simulink model "Power_Systems_II_Simulation"  (R2022b)
settings: Solver=VariableStepAuto  StartTime=0.0  StopTime=4  RelTol=1e-3
libraries: spsGroundLib x5, spsVoltageMeasurementLib x3, spsThreePhaseFaultLib x1, spsCurrentMeasurementLib x1, spsDistributedParametersLineLib x1, spsThreePhaseSeriesRLCBranchLib x1, spsThreePhaseSourceLib x1, sps_lib x1
settings Model: Creator=USER  LastModifiedBy=USER

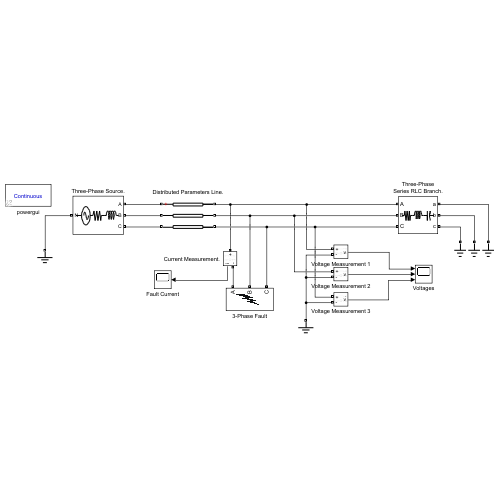
[thumbnail: Simulink's stored preview of the top-level diagram]
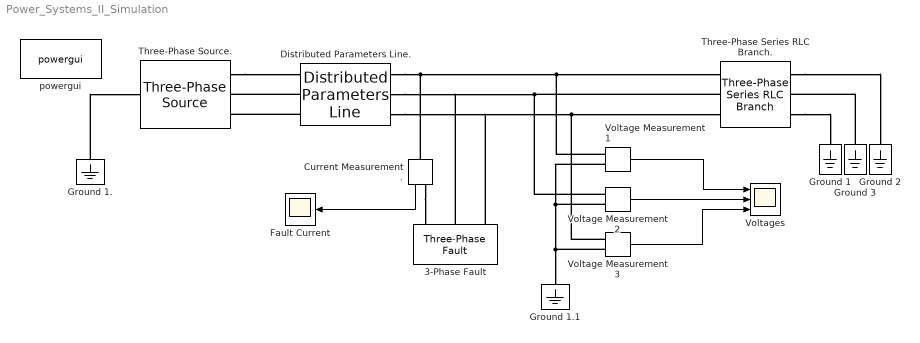
== system Power_Systems_II_Simulation ==
  3-Phase Fault : spsThreePhaseFaultLib/Three-Phase Fault  InitialStates=1  FaultA=on  FaultB=off  FaultC=off  GroundFault=on  SwitchTimes="[1  5]"  External=off  SwitchStatus=NaN  FaultResistance=0.01  GroundResistance=0.01  SnubberResistance=1e6  SnubberCapacitance=inf  Measurements=None
  Current Measurement. : spsCurrentMeasurementLib/Current Measurement  PhasorSimulation=off  OutputType=Complex  PSBequivalent=0
  Distributed Parameters Line. : spsDistributedParametersLineLib/Distributed Parameters Line  Phases=3  Length=10  Frequency=50  Resistance=[0.1 0.1]  Inductance=[0.3183 0.00095]  Capacitance=[0.00001 0.00001]  x1=[77.8287131632967 10973.8048950639 11040.6367185842;314.159265358979 314.159265358979 314.159265358979;-1.71456896003776 1.19594865444981 -0.369209675509595]  x2=[281.416313881128 4968.77740365391 8364.21694231392;314.159265358979 314.159265358979 314.159265358979;-0.928264752183291 2.28039663965508 -0.898944896122367]  x3=[78.9240246113386 59.1908510089468 99.800748397703;314.159265358979 314.159265358979 314.159265358979;-1.9368174494414 -0.00240562107416638 -0.495420267168485]  x4=[57.5363481374095 114.643353425724 27.3819360505492;314.159265358979 314.159265358979 314.159265358979;0.834085976351815 2.37283316623951 0.779404320473407]  x5=0.0178409640995099  V1=[77.83 1.097e+04 1.104e+04;314.2 314.2 314.2;-1.715 1.196 -0.3692]  V2=[281.4 4969 8364;314.2 314.2 314.2;-0.9283 2.28 -0.8989]  I1=[78.92 59.19 99.8;314.2 314.2 314.2;-1.937 -0.002406 -0.4954]  I2=[57.54 114.6 27.38;314.2 314.2 314.2;0.8341 2.373 0.7794]  nHarmo=1  Measurements=None  Decoupling=off  VsMag0=0  VrMag0=0  VsAngle0=0  VrAngle0=0  IsMag0=0  IrMag0=0  IsAngle0=0  IrAngle0=0
      settings: LibrarySourceBlock=sps_lib/Power Grid Elements/Distributed Parameters Line
  Fault Current : Scope
  Ground 1 : spsGroundLib/Ground  LConnTagsString=a
  Ground 1. : spsGroundLib/Ground  LConnTagsString=a
  Ground 1.1 : spsGroundLib/Ground  LConnTagsString=a
  Ground 2 : spsGroundLib/Ground  LConnTagsString=a
  Ground 3 : spsGroundLib/Ground  LConnTagsString=a
  Three-Phase Series RLC Branch. : spsThreePhaseSeriesRLCBranchLib/Three-Phase Series RLC Branch  LConnTagsString=A|B|C  RConnTagsString=A|B|C  BranchType=RLC  Resistance=3  Inductance=0.000795774  Capacitance=0.00001  Measurements=None
  Three-Phase Source. : spsThreePhaseSourceLib/Three-Phase Source  InternalConnection=Yn  VoltagePhases=off  Voltage=11000  PhaseAngle=0  Voltage_phases=[25e3 25e3 25e3]/sqrt(3)  PhaseAngles_phases=[0 -120 +120]  Frequency=50  NonIdealSource=on  SpecifyImpedance=off  Resistance=1  Inductance=0.000795774  ShortCircuitLevel=100e6  BaseVoltage=11000  XRratio=7  BusType=swing  Pref=10e3  Qref=0  Prefabc=[10e3, 10e3, 10e3]  Qrefabc=[0, 0, 0]  Qmin=-inf  Qmax=inf
  Voltage Measurement 1 : spsVoltageMeasurementLib/Voltage Measurement  PhasorSimulation=off  OutputType=Complex  PSBequivalent=0
  Voltage Measurement 2 : spsVoltageMeasurementLib/Voltage Measurement  PhasorSimulation=off  OutputType=Complex  PSBequivalent=0
  Voltage Measurement 3 : spsVoltageMeasurementLib/Voltage Measurement  PhasorSimulation=off  OutputType=Complex  PSBequivalent=0
  Voltages : Scope  NumInputPorts=3
  powergui : sps_lib/powergui  Priority=1  SimulationMode=Continuous  SampleTime=50e-6  frequency=60  Iterations=50  frequencyindice=50  Pbase=100e6  ErrMax=1e-4  UnitsV=kV  UnitsW=MW  buscounter=0  FunctionMessages=off  echomessages=off  EnableUseOfTLC=off  CurrentSourceSwitches=off  DisableSnubberDevices=off  DisableRonSwitches=off  DisableVfSwitches=off  DisplayEquations=off  AutomaticDiscreteSolvers=off  SolverType=Tustin/Backward Euler (TBE)  Interpol=off  ExternalGateDelay=off  methode=off  Ts=100  x0status=blocks  SPID=on  SwTol=0  HookPort=off  NonlinearTolerance=1e-4  nMaxIteration=100  ContinueOnMaxIteration=off  RestoreLinks=warning  ResistiveCurrentMeasurement=off  Frange=[0:2:500]  Ylog=off  Xlog=on  ShowGrid=off  save=off  variable=ZData  structure=0  ZoomFFT=off  StartTime=0.0  cycles=1  DisplayStyle=1  fundamental=60  FreqAxis=off  MaxFrequency=1000  frequencyindicesteady=1  RmsSteady=1  display=off
  wires:
  Voltage Measurement 1/1 -> Voltages/1
  Voltage Measurement 2/1 -> Voltages/2
  Voltage Measurement 3/1 -> Voltages/3
  Current Measurement./1 -> Fault Current/1
  connections:
  Three-Phase Source./RConn1 -- Distributed Parameters Line./LConn1
  Ground 1./LConn1 -- Three-Phase Source./LConn1
  Distributed Parameters Line./LConn3 -- Three-Phase Source./RConn3
  Distributed Parameters Line./LConn2 -- Three-Phase Source./RConn2
  Distributed Parameters Line./RConn1 -- Current Measurement./LConn1 -- Voltage Measurement 1/LConn1 -- Three-Phase Series RLC Branch./LConn1
  Three-Phase Series RLC Branch./LConn2 -- Distributed Parameters Line./RConn2 -- 3-Phase Fault/LConn2 -- Voltage Measurement 2/LConn1
  Voltage Measurement 3/LConn1 -- Distributed Parameters Line./RConn3 -- 3-Phase Fault/LConn3 -- Three-Phase Series RLC Branch./LConn3
  Voltage Measurement 1/LConn2 -- Voltage Measurement 2/LConn2 -- Voltage Measurement 3/LConn2 -- Ground 1.1/LConn1
  Ground 3/LConn1 -- Three-Phase Series RLC Branch./RConn2
  Three-Phase Series RLC Branch./RConn3 -- Ground 1/LConn1
  Three-Phase Series RLC Branch./RConn1 -- Ground 2/LConn1
  Current Measurement./RConn1 -- 3-Phase Fault/LConn1
